simulink model "Hypnoz_embedded_continu_v008"  (Simulink 7.7)
settings: Solver=ode3  StartTime=0.0  StopTime=50  FixedStep=Ts  RelTol=1e-3
values from neighbouring files (symbols this model uses):
  A = [-r/L -k/L;km/J -lambda/J]    [SimulationParams.m]
  B = [1/L;0]    [SimulationParams.m]
  Coeff_reprise_obs_I = 1    [SimulationParams.m]
  Coeff_reprise_obs_U = 1    [SimulationParams.m]
  Cs = 196/4    (= 49)    [SimulationParams.m]
  Delt_I2t_max = 1000    [SimulationParams.m]
  Delt_Imot_max = 5    [SimulationParams.m]
  Delt_U2t_max = 1000    [SimulationParams.m]
  Delt_Umot_max = 5    [SimulationParams.m]
  I2t_max = 200000    [SimulationParams.m]
  Imot_max = 220    [SimulationParams.m]
  Isc_max = 300    [SimulationParams.m]
  k = 1/52    (= 0.0192307692308)    [SimulationParams.m]
  Ka = place(Aa,Ba,[p1 p2 p3])    [SimulationParams.m]
  km = 0.16    [SimulationParams.m]
  Koi = K(3:4,:)    [SimulationParams.m]
  Kop = K(1:2,:)    [SimulationParams.m]
  L = 53E-6    (= 5.3e-05)    [SimulationParams.m]
  Masse_vehicule = 850    [SimulationParams.m]
  Pmax_boost = 11750    [SimulationParams.m]
  Pmax_brake = 25000    [SimulationParams.m]
  r = 0.0175    [SimulationParams.m]
  rapport_vitesses = empatement/Rayon_braquage    (= 0.15)    [SimulationParams.m]
  rayon_roue = 0.31    [SimulationParams.m]
  Reduction_electrique = 1/3    (= 0.333333333333)    [SimulationParams.m]
  Th_down = -5    [SimulationParams.m]
  Th_up = 90    [SimulationParams.m]
  to = 0.03    [SimulationParams.m]
  Tr1 = 1000    [SimulationParams.m]
  Tr2 = 1000    [SimulationParams.m]
  Tr6 = 1/Ts    (= 1000)    [SimulationParams.m]
  Ts = 0.001    [SimulationParams.m]
  Ts_sc = 0.005    [SimulationParams.m]
  Umot_max = 96    [SimulationParams.m]
  Usc_max = 192    [SimulationParams.m]
  Usc_min = 96    [SimulationParams.m]
undefined symbols (not defined in the file or in its folder): sigbuilder_block
libraries: simulink x10, simulink_extras x1
(part 1 of 2)
settings Model: Creator=F.NICOLAS  LastModifiedBy=Guilherme  BufferReuse=off
settings DataIOCC: SaveOutput=off  SignalLogging=off  SaveTime=off
settings OptimizationCC: BlockReduction=off  BooleanDataType=off  OptimizeBlockIOStorage=off  BufferReuse=off  ExpressionFolding=off  LocalBlockOutputs=off  InitFltsAndDblsToZero=on
settings DebuggingCC: ArtificialAlgebraicLoopMsg=error  SaveWithParameterizedLinksMsg=none  SignalResolutionControl=TryResolveAllWithWarning  MultiTaskCondExecSysMsg=none  StrictBusMsg=Warning
settings HardwareCC: ProdHWDeviceType=Generic->Unspecified (assume 32-bit Generic)
settings SFSimCC: SimParseCustomCode=off
settings RTWCC: IncludeERTFirstTime=on
settings GRTTargetCC: TargetFcnLib=ansi_tfl_tmw.mat

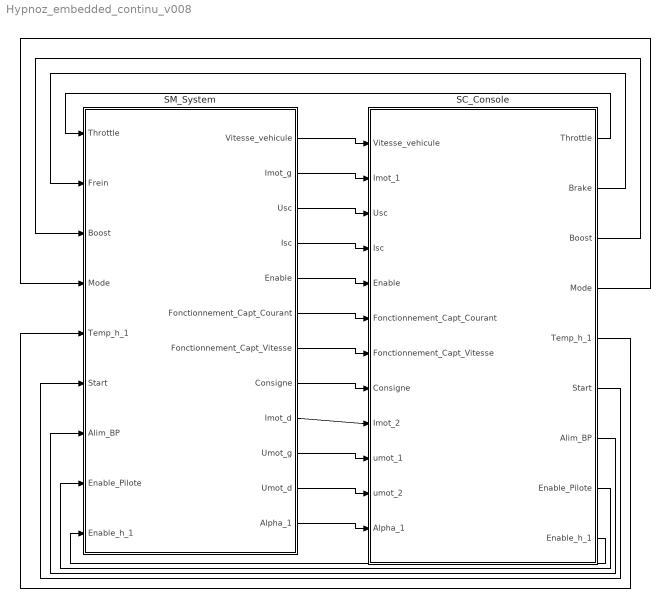
== system Hypnoz_embedded_continu_v008 ==
  SC_Console : Subsystem
  SM_System : Subsystem
  wires:
  SC_Console/1(Throttle) -> SM_System/1(Throttle)
  SC_Console/3(Boost) -> SM_System/3(Boost)
  SM_System/1(Vitesse_vehicule) -> SC_Console/1(Vitesse_vehicule)
  SC_Console/4(Mode) -> SM_System/4(Mode)
  SC_Console/2(Brake) -> SM_System/2(Frein)
  SM_System/2(Imot_g) -> SC_Console/2(Imot_1)
  SM_System/3(Usc) -> SC_Console/3(Usc)
  SM_System/4(Isc) -> SC_Console/4(Isc)
  SM_System/5(Enable) -> SC_Console/5(Enable)
  SM_System/6(Fonctionnement_Capt_Courant) -> SC_Console/6(Fonctionnement_Capt_Courant)
  SM_System/8(Consigne) -> SC_Console/8(Consigne)
  SM_System/9(Imot_d) -> SC_Console/9(Imot_2)
  SM_System/10(Umot_g) -> SC_Console/10(umot_1)
  SM_System/11(Umot_d) -> SC_Console/11(umot_2)
  SM_System/7(Fonctionnement_Capt_Vitesse) -> SC_Console/7(Fonctionnement_Capt_Vitesse)
  SC_Console/9(Enable_h_1) -> SM_System/9(Enable_h_1)
  SC_Console/8(Enable_Pilote) -> SM_System/8(Enable_Pilote)
  SC_Console/7(Alim_BP) -> SM_System/7(Alim_BP)
  SC_Console/6(Start) -> SM_System/6(Start)
  SC_Console/5(Temp_h_1) -> SM_System/5(Temp_h_1)
  SM_System/12(Alpha_1) -> SC_Console/12(Alpha_1)

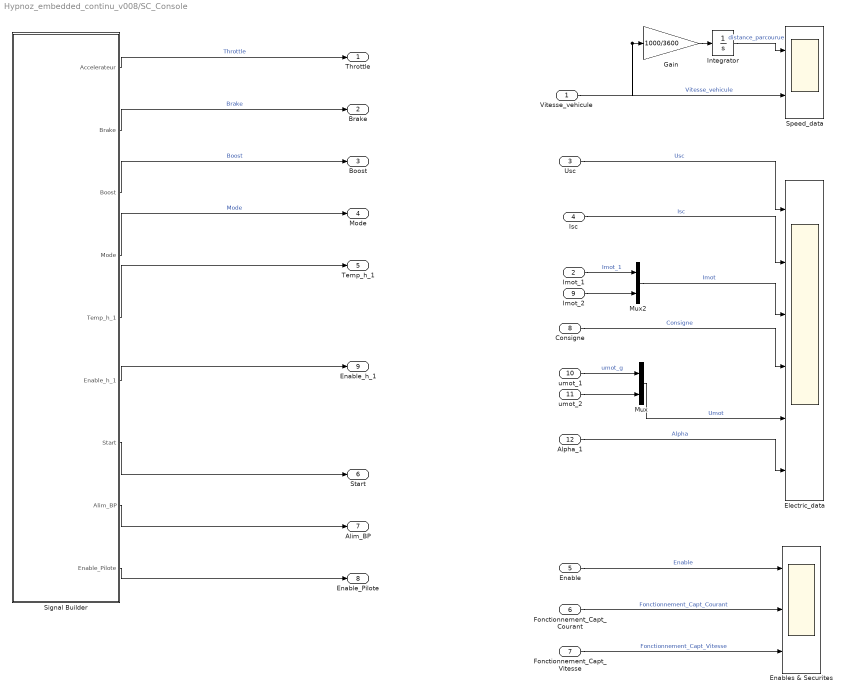
== system Hypnoz_embedded_continu_v008/SC_Console ==
  Vitesse_vehicule : Inport
  Imot_1 : Inport  Port=2
  Usc : Inport  Port=3
  Isc : Inport  Port=4
  Enable : Inport  Port=5
  Fonctionnement_Capt_Courant : Inport  Port=6
  Fonctionnement_Capt_Vitesse : Inport  Port=7
  Consigne : Inport  Port=8
  Imot_2 : Inport  Port=9
  umot_1 : Inport  Port=10
  umot_2 : Inport  Port=11
  Alpha_1 : Inport  Port=12
  Electric_data : Scope  NumInputPorts=6
      settings: TimeRange=4  YMin=149.1~-9~55~0~0.5~0.01  YMax=150~-1~100~100~5~0.045  SaveName=ScopeData21
  Enables & Securites : Scope  NumInputPorts=3
      settings: YMin=0.95~0.95~0.95  YMax=1.05~1.05~1.05
  Gain : Gain  Gain=1000/3600
  Integrator : Integrator
  Mux : Mux  Inputs=2
  Mux2 : Mux  Inputs=2
  Signal Builder : Subsystem  Tag=STV Subsys  LoadFcn=sigbuilder_block('load');  StartFcn=sigbuilder_block('start');  StopFcn=sigbuilder_block('stop');  ClipboardFcn=sigbuilder_block('clipboard');  mask(Sigbuilder block){}
      mask help: Sigbuilder GUI
      mask init:
      | if ~strcmp(get_param(bdroot(gcbh),'SimulationStatus'),'stopped') tuvar = sigbuilder_block('maskInit'); end
      settings: CopyFcn=sigbuilder_block('copy');  DeleteFcn=sigbuilder_block('delete');  ModelCloseFcn=sigbuilder_block('modelClose');  PreSaveFcn=sigbuilder_block('preSave');  NameChangeFcn=sigbuilder_block('namechange');  OpenFcn=sigbuilder_block('open',[6 21 1012.5 492 ]);  CloseFcn=sigbuilder_block('close');
      mask Display: plot(0,0,100,100,[10,10,40,40,10],[80,20,20,80,80],[40,10],[50,50], [40,27,10],[65,72,56],[40,25,25,10],[28,28,43,43]);
  Speed_data : Scope  NumInputPorts=2
      settings: TimeRange=4  YMin=10~27.5  YMax=90~52.5
  Throttle : Outport
  Brake : Outport  Port=2
  Boost : Outport  Port=3
  Mode : Outport  Port=4
  Temp_h_1 : Outport  Port=5
  Start : Outport  Port=6
  Alim_BP : Outport  Port=7
  Enable_Pilote : Outport  Port=8
  Enable_h_1 : Outport  Port=9
  wires:
  Signal Builder/1(Accelerateur) -> Throttle/1  "Throttle"
  Vitesse_vehicule/1 -> Gain/1, Speed_data/2  "Vitesse_vehicule"
  Signal Builder/2(Brake) -> Brake/1  "Brake"
  Signal Builder/3(Boost) -> Boost/1  "Boost"
  Signal Builder/4(Mode) -> Mode/1  "Mode"
  Gain/1 -> Integrator/1
  Integrator/1 -> Speed_data/1  "distance_parcourue"
  Usc/1 -> Electric_data/1  "Usc"
  Isc/1 -> Electric_data/2  "Isc"
  Signal Builder/5(Temp_h_1) -> Temp_h_1/1
  Consigne/1 -> Electric_data/4  "Consigne"
  Signal Builder/6(Enable_h_1) -> Enable_h_1/1
  Signal Builder/7(Start) -> Start/1
  Signal Builder/8(Alim_BP) -> Alim_BP/1
  Signal Builder/9(Enable_Pilote) -> Enable_Pilote/1
  Imot_1/1 -> Mux2/1  "Imot_1"
  Enable/1 -> Enables & Securites/1  "Enable"
  Fonctionnement_Capt_Courant/1 -> Enables & Securites/2  "Fonctionnement_Capt_Courant"
  Fonctionnement_Capt_Vitesse/1 -> Enables & Securites/3  "Fonctionnement_Capt_Vitesse"
  Mux/1 -> Electric_data/5  "Umot"
  umot_1/1 -> Mux/1  "umot_g"
  Alpha_1/1 -> Electric_data/6  "Alpha"
  umot_2/1 -> Mux/2
  Mux2/1 -> Electric_data/3  "Imot"
  Imot_2/1 -> Mux2/2

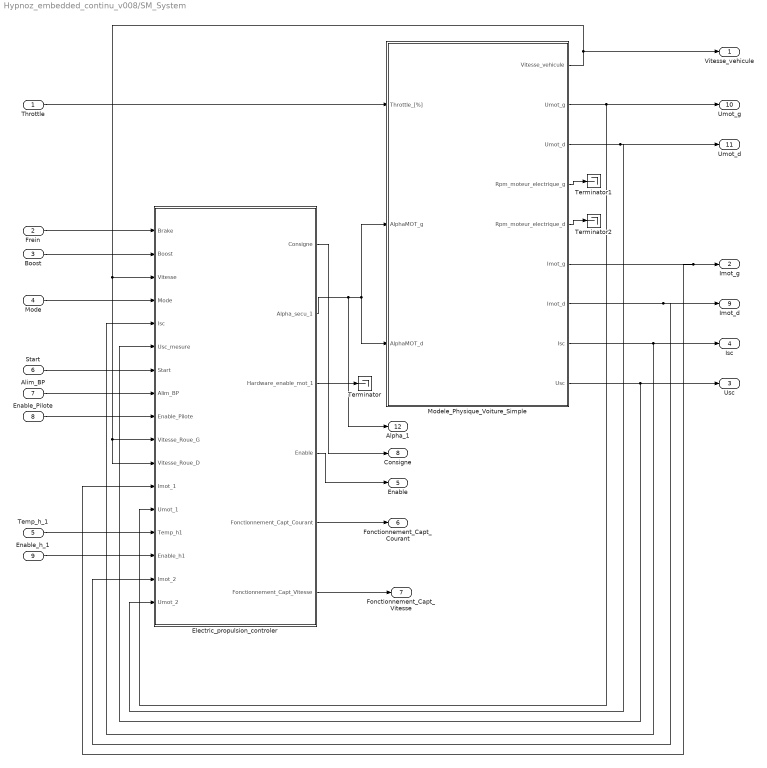
== system Hypnoz_embedded_continu_v008/SM_System ==
  Throttle : Inport
  Frein : Inport  Port=2
  Boost : Inport  Port=3
  Mode : Inport  Port=4
  Temp_h_1 : Inport  Port=5
  Start : Inport  Port=6
  Alim_BP : Inport  Port=7
  Enable_Pilote : Inport  Port=8
  Enable_h_1 : Inport  Port=9
  Electric_propulsion_controler : Subsystem
  Modele_Physique_Voiture_Simple : Subsystem
  Terminator : Terminator
  Terminator1 : Terminator
  Terminator2 : Terminator
  Vitesse_vehicule : Outport
  Imot_g : Outport  Port=2
  Usc : Outport  Port=3
  Isc : Outport  Port=4
  Enable : Outport  Port=5
  Fonctionnement_Capt_Courant : Outport  Port=6
  Fonctionnement_Capt_Vitesse : Outport  Port=7
  Consigne : Outport  Port=8
  Imot_d : Outport  Port=9
  Umot_g : Outport  Port=10
  Umot_d : Outport  Port=11
  Alpha_1 : Outport  Port=12
  wires:
  Modele_Physique_Voiture_Simple/1(Vitesse_vehicule) -> Vitesse_vehicule/1, Electric_propulsion_controler/3(Vitesse), Electric_propulsion_controler/10(Vitesse_Roue_G), Electric_propulsion_controler/11(Vitesse_Roue_D)
  Boost/1 -> Electric_propulsion_controler/2(Boost)
  Mode/1 -> Electric_propulsion_controler/4(Mode)
  Electric_propulsion_controler/4(Enable) -> Enable/1
  Electric_propulsion_controler/1(Consigne) -> Consigne/1
  Modele_Physique_Voiture_Simple/6(Imot_g) -> Imot_g/1, Electric_propulsion_controler/12(Imot_1)
  Modele_Physique_Voiture_Simple/7(Imot_d) -> Imot_d/1, Electric_propulsion_controler/16(Imot_2)
  Modele_Physique_Voiture_Simple/8(Isc) -> Isc/1, Electric_propulsion_controler/5(Isc)
  Frein/1 -> Electric_propulsion_controler/1(Brake)
  Modele_Physique_Voiture_Simple/9(Usc) -> Usc/1, Electric_propulsion_controler/6(Usc_mesure)
  Modele_Physique_Voiture_Simple/3(Umot_d) -> Umot_d/1, Electric_propulsion_controler/17(Umot_2)
  Modele_Physique_Voiture_Simple/2(Umot_g) -> Umot_g/1, Electric_propulsion_controler/13(Umot_1)
  Electric_propulsion_controler/2(Alpha_secu_1) -> Alpha_1/1, Modele_Physique_Voiture_Simple/2(AlphaMOT_g), Modele_Physique_Voiture_Simple/3(AlphaMOT_d)
  Electric_propulsion_controler/5(Fonctionnement_Capt_Courant) -> Fonctionnement_Capt_Courant/1
  Electric_propulsion_controler/6(Fonctionnement_Capt_Vitesse) -> Fonctionnement_Capt_Vitesse/1
  Temp_h_1/1 -> Electric_propulsion_controler/14(Temp_h1)
  Start/1 -> Electric_propulsion_controler/7(Start)
  Alim_BP/1 -> Electric_propulsion_controler/8(Alim_BP)
  Enable_Pilote/1 -> Electric_propulsion_controler/9(Enable_Pilote)
  Enable_h_1/1 -> Electric_propulsion_controler/15(Enable_h1)
  Throttle/1 -> Modele_Physique_Voiture_Simple/1(Throttle_[%])
  Electric_propulsion_controler/3(Hardware_enable_mot_1) -> Terminator/1
  Modele_Physique_Voiture_Simple/4(Rpm_moteur_electrique_g) -> Terminator1/1
  Modele_Physique_Voiture_Simple/5(Rpm_moteur_electrique_d) -> Terminator2/1

== system Hypnoz_embedded_continu_v008/SC_Console/Signal Builder ==
  Demux : Demux  Tag=STV Demux  Outputs=9
  FromWs : FromWorkspace  Tag=STV FromWs  VariableName=tuvar  SampleTime=0  SigBuilderData=DataTag0  VnvData=DataTag1
      SigBuilderData=|
      | common.afterFinalStr = 'Extrapolate'
      | common.sampleTime = 0
      | dataSet.timeRange = [0 40]
      | dataSet.name = 'Group 1'
      | sbobj.Groups(1).Name = 'Group 1'
      | sbobj.Groups(1).Signals(1).Name = 'Accelerateur'
      | sbobj.Groups(1).Signals(1).XData = [0 40]
      | sbobj.Groups(1).Signals(1).YData = [0 0]
      | sbobj.Groups(1).Signals(2).Name = 'Brake'
      | sbobj.Groups(1).Signals(2).XData = [0 1.57 2.48 5.39 5.82 20 20 30 30 40]
      | sbobj.Groups(1).Signals(2).YData = [0 0 0 0 0 0 0.95 0.95 0 0]
      | sbobj.Groups(1).Signals(3).Name = 'Boost'
      | sbobj.Groups(1).Signals(3).XData = [0 5 10 15 15 20 25 30 35 40]
      | sbobj.Groups(1).Signals(3).YData = [0 0 1 1 0 0 0 0 0 0]
      | sbobj.Groups(1).Signals(4).Name = 'Mode'
      | sbobj.Groups(1).Signals(4).XData = [0 40]
      | sbobj.Groups(1).Signals(4).YData = [2 2]
      | sbobj.Groups(1).Signals(5).Name = 'Temp_h_1'
      | sbobj.Groups(1).Signals(5).XData = [0 40]
      | sbobj.Groups(1).Signals(5).YData = [60 60]
      | sbobj.Groups(1).Signals(6).Name = 'Enable_h_1'
      | sbobj.Groups(1).Signals(6).XData = [0 40]
      | sbobj.Groups(1).Signals(6).YData = [1 1]
      | sbobj.Groups(1).Signals(7).Name = 'Start'
      | sbobj.Groups(1).Signals(7).XData = [0 1 1 2 2 40]
      | sbobj.Groups(1).Signals(7).YData = [0 0 1 1 0 0]
      | sbobj.Groups(1).Signals(8).Name = 'Alim_BP'
      | sbobj.Groups(1).Signals(8).XData = [0 40]
      | sbobj.Groups(1).Signals(8).YData = [1 1]
      | sbobj.Groups(1).Signals(9).Name = 'Enable_Pilote'
      | sbobj.Groups(1).Signals(9).XData = [0 40]
      | sbobj.Groups(1).Signals(9).YData = [1 1]
      | sbobj.Groups(1).TimeRange = [0 40]
      | sbobj.Groups(2).Name = 'Group 2'
      | sbobj.Groups(2).Signals(1).Name = 'Accelerateur'
      | sbobj.Groups(2).Signals(1).XData = [0 100]
      | sbobj.Groups(2).Signals(1).YData = [0 0]
      | sbobj.Groups(2).Signals(2).Name = 'Brake'
      | sbobj.Groups(2).Signals(2).XData = [0 1.57 2.48 5.39 5.82 19.1 27.1 100]
      | sbobj.Groups(2).Signals(2).YData = [0 0 0 0 0 0 0 0]
      | sbobj.Groups(2).Signals(3).Name = 'Boost'
      | sbobj.Groups(2).Signals(3).XData = [0 10 20 20 30 30 40 40 50 50 60 60 70 70 80 80 90 90 100]
      | sbobj.Groups(2).Signals(3).YData = [0 0 2 0 2 0 2 0 2 0 2 0 2 0 2 0 2 0 2]
      | sbobj.Groups(2).Signals(4).Name = 'Mode'
      | sbobj.Groups(2).Signals(4).XData = [0 100]
      | sbobj.Groups(2).Signals(4).YData = [2 2]
      | sbobj.Groups(2).Signals(5).Name = 'Temp_h_1'
      | sbobj.Groups(2).Signals(5).XData = [0 100]
      | sbobj.Groups(2).Signals(5).YData = [60 60]
      | sbobj.Groups(2).Signals(6).Name = 'Enable_h_1'
      | sbobj.Groups(2).Signals(6).XData = [0 100]
      | sbobj.Groups(2).Signals(6).YData = [1 1]
      | sbobj.Groups(2).Signals(7).Name = 'Start'
      | sbobj.Groups(2).Signals(7).XData = [0 1 1 2 2 100]
      | sbobj.Groups(2).Signals(7).YData = [0 0 1 1 0 0]
      | sbobj.Groups(2).Signals(8).Name = 'Alim_BP'
      | sbobj.Groups(2).Signals(8).XData = [0 100]
      | sbobj.Groups(2).Signals(8).YData = [1 1]
      | sbobj.Groups(2).Signals(9).Name = 'Enable_Pilote'
      | sbobj.Groups(2).Signals(9).XData = [0 100]
      | sbobj.Groups(2).Signals(9).YData = [1 1]
  Accelerateur : Outport  Tag=STV Outport
  Brake : Outport  Tag=STV Outport  Port=2
  Boost : Outport  Tag=STV Outport  Port=3
  Mode : Outport  Tag=STV Outport  Port=4
  Temp_h_1 : Outport  Tag=STV Outport  Port=5
  Enable_h_1 : Outport  Tag=STV Outport  Port=6
  Start : Outport  Tag=STV Outport  Port=7
  Alim_BP : Outport  Tag=STV Outport  Port=8
  Enable_Pilote : Outport  Tag=STV Outport  Port=9
  wires:
  FromWs/1 -> Demux/1
  Demux/1 -> Accelerateur/1
  Demux/2 -> Brake/1
  Demux/3 -> Boost/1
  Demux/4 -> Mode/1
  Demux/5 -> Temp_h_1/1
  Demux/6 -> Enable_h_1/1
  Demux/7 -> Start/1
  Demux/8 -> Alim_BP/1
  Demux/9 -> Enable_Pilote/1

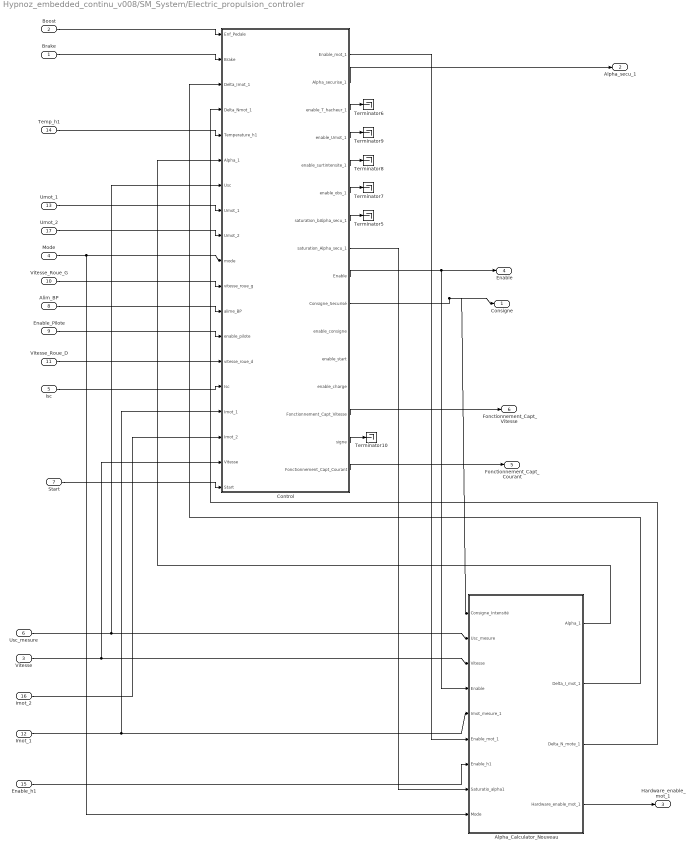
== system Hypnoz_embedded_continu_v008/SM_System/Electric_propulsion_controler ==
  Brake : Inport
  Boost : Inport  Port=2
  Vitesse : Inport  Port=3
  Mode : Inport  Port=4
  Isc : Inport  Port=5
  Usc_mesure : Inport  Port=6
  Start : Inport  Port=7
  Alim_BP : Inport  Port=8
  Enable_Pilote : Inport  Port=9
  Vitesse_Roue_G : Inport  Port=10
  Vitesse_Roue_D : Inport  Port=11
  Imot_1 : Inport  Port=12
  Umot_1 : Inport  Port=13
  Temp_h1 : Inport  Port=14
  Enable_h1 : Inport  Port=15
  Imot_2 : Inport  Port=16
  Umot_2 : Inport  Port=17
  Alpha_Calculator_Nouveau : Subsystem
  Control : Subsystem
  Terminator{5..10} (6 alike) : Terminator
  Consigne : Outport
  Alpha_secu_1 : Outport  Port=2
  Hardware_enable_mot_1 : Outport  Port=3
  Enable : Outport  Port=4
  Fonctionnement_Capt_Courant : Outport  Port=5
  Fonctionnement_Capt_Vitesse : Outport  Port=6
  wires:
  Control/10(Consigne_Securisé) -> Alpha_Calculator_Nouveau/1(Consigne_Intensité), Consigne/1
  Alpha_Calculator_Nouveau/1(Alpha_1) -> Control/6(Alpha_1)
  Boost/1 -> Control/1(Enf_Pedale)
  Brake/1 -> Control/2(Brake)
  Control/9(Enable) -> Alpha_Calculator_Nouveau/4(Enable), Enable/1
  Control/1(Enable_mot_1) -> Alpha_Calculator_Nouveau/6(Enable_mot_1)
  Mode/1 -> Control/10(mode), Alpha_Calculator_Nouveau/9(Mode)
  Usc_mesure/1 -> Alpha_Calculator_Nouveau/2(Usc_mesure), Control/7(Usc)
  Imot_1/1 -> Alpha_Calculator_Nouveau/5(Imot_mesure_1), Control/16(Imot_1)
  Imot_2/1 -> Control/17(Imot_2)
  Isc/1 -> Control/15(Isc)
  Vitesse/1 -> Alpha_Calculator_Nouveau/3(Vitesse), Control/18(Vitesse)
  Enable_h1/1 -> Alpha_Calculator_Nouveau/7(Enable_h1)
  Control/8(saturation_Alpha_secu_1) -> Alpha_Calculator_Nouveau/8(Saturatio_alpha1)
  Control/7(saturation_bAlpha_secu_1) -> Terminator5/1
  Control/6(enable_obs_1) -> Terminator7/1
  Control/5(enable_surtintensite_1) -> Terminator8/1
  Control/4(enable_Umot_1) -> Terminator9/1
  Control/3(enable_T_hacheur_1) -> Terminator6/1
  Temp_h1/1 -> Control/5(Temperature_h1)
  Umot_2/1 -> Control/9(Umot_2)
  Umot_1/1 -> Control/8(Umot_1)
  Vitesse_Roue_D/1 -> Control/14(vitesse_roue_d)
  Vitesse_Roue_G/1 -> Control/11(vitesse_roue_g)
  Start/1 -> Control/19(Start)
  Enable_Pilote/1 -> Control/13(enable_pilote)
  Alim_BP/1 -> Control/12(alime_BP)
  Alpha_Calculator_Nouveau/2(Delta_I_mot_1) -> Control/3(Delta_Imot_1)
  Alpha_Calculator_Nouveau/3(Delta_N_mote_1) -> Control/4(Delta_Nmot_1)
  Control/2(Alpha_securise_1) -> Alpha_secu_1/1
  Alpha_Calculator_Nouveau/4(Hardware_enable_mot_1) -> Hardware_enable_mot_1/1
  Control/16(Fonctionnement_Capt_Courant) -> Fonctionnement_Capt_Courant/1
  Control/14(Fonctionnement_Capt_Vitesse) -> Fonctionnement_Capt_Vitesse/1
  Control/15(signe) -> Terminator10/1

== system Hypnoz_embedded_continu_v008/SM_System/Modele_Physique_Voiture_Simple ==
  Throttle_[%] : Inport
  AlphaMOT_g : Inport  Port=2
  AlphaMOT_d : Inport  Port=3
  Circuit_electrique_HP : Subsystem
  Couple_Max : Gain  Gain=130
  Modèle_Simplifiè Véhicule : Subsystem
  Terminator : Terminator
  Vitesse_vehicule : Outport
  Umot_g : Outport  Port=2
  Umot_d : Outport  Port=3
  Rpm_moteur_electrique_g : Outport  Port=4
  Rpm_moteur_electrique_d : Outport  Port=5
  Imot_g : Outport  Port=6
  Imot_d : Outport  Port=7
  Isc : Outport  Port=8
  Usc : Outport  Port=9
  wires:
  Circuit_electrique_HP/2(I Mot_d) -> Imot_d/1, Modèle_Simplifiè Véhicule/3(Imot_d)
  AlphaMOT_g/1 -> Circuit_electrique_HP/3(AlphaMOT_g)
  AlphaMOT_d/1 -> Circuit_electrique_HP/4(AlphaMOT_d)
  Circuit_electrique_HP/3(Isc) -> Isc/1
  Circuit_electrique_HP/4(Usc) -> Usc/1
  Circuit_electrique_HP/5(Umot_g) -> Umot_g/1
  Circuit_electrique_HP/6(Umot_d) -> Umot_d/1
  Circuit_electrique_HP/1(I Mot_g) -> Imot_g/1, Modèle_Simplifiè Véhicule/2(Imot_g)
  Throttle_[%]/1 -> Couple_Max/1
  Couple_Max/1 -> Modèle_Simplifiè Véhicule/1(Couple_thermique)
  Modèle_Simplifiè Véhicule/2(Vitesse_Vehicule) -> Vitesse_vehicule/1
  Modèle_Simplifiè Véhicule/3(RPM_Moteur_Electrique) -> Rpm_moteur_electrique_g/1, Circuit_electrique_HP/1(Rpm_moteur_electrique_g), Rpm_moteur_electrique_d/1, Circuit_electrique_HP/2(Rpm_moteur_electrique_d)
  Modèle_Simplifiè Véhicule/1(couple_roue) -> Terminator/1

== system Hypnoz_embedded_continu_v008/SM_System/Electric_propulsion_controler/Alpha_Calculator_Nouveau ==
  Consigne_Intensité : Inport
  Usc_mesure : Inport  Port=2
  Vitesse : Inport  Port=3
  Enable : Inport  Port=4
  Imot_mesure_1 : Inport  Port=5
  Enable_mot_1 : Inport  Port=6
  Enable_h1 : Inport  Port=7
  Saturatio_alpha1 : Inport  Port=8
  Mode : Inport  Port=9
  Alpha_calculator_motg1 : Subsystem
  Alpha_1 : Outport
  Delta_I_mot_1 : Outport  Port=2
  Delta_N_mote_1 : Outport  Port=3
  Hardware_enable_mot_1 : Outport  Port=4
  wires:
  Consigne_Intensité/1 -> Alpha_calculator_motg1/1(Consigne_intensité)
  Alpha_calculator_motg1/1(Alpha_g) -> Alpha_1/1
  Imot_mesure_1/1 -> Alpha_calculator_motg1/2(Imot_mesure_g)
  Usc_mesure/1 -> Alpha_calculator_motg1/3(Usc_mesure)
  Alpha_calculator_motg1/2(Delta_I_mot_g1) -> Delta_I_mot_1/1
  Vitesse/1 -> Alpha_calculator_motg1/4(Vitesse)
  Enable/1 -> Alpha_calculator_motg1/5(enable)
  Enable_mot_1/1 -> Alpha_calculator_motg1/6(enable_mot_g1)
  Alpha_calculator_motg1/3(Delta_N_mot_g1) -> Delta_N_mote_1/1
  Saturatio_alpha1/1 -> Alpha_calculator_motg1/8(Saturation_alpha1)
  Alpha_calculator_motg1/4(Hardware_enable_mot_1) -> Hardware_enable_mot_1/1
  Enable_h1/1 -> Alpha_calculator_motg1/7(enable_h1)
  Mode/1 -> Alpha_calculator_motg1/9(mode)

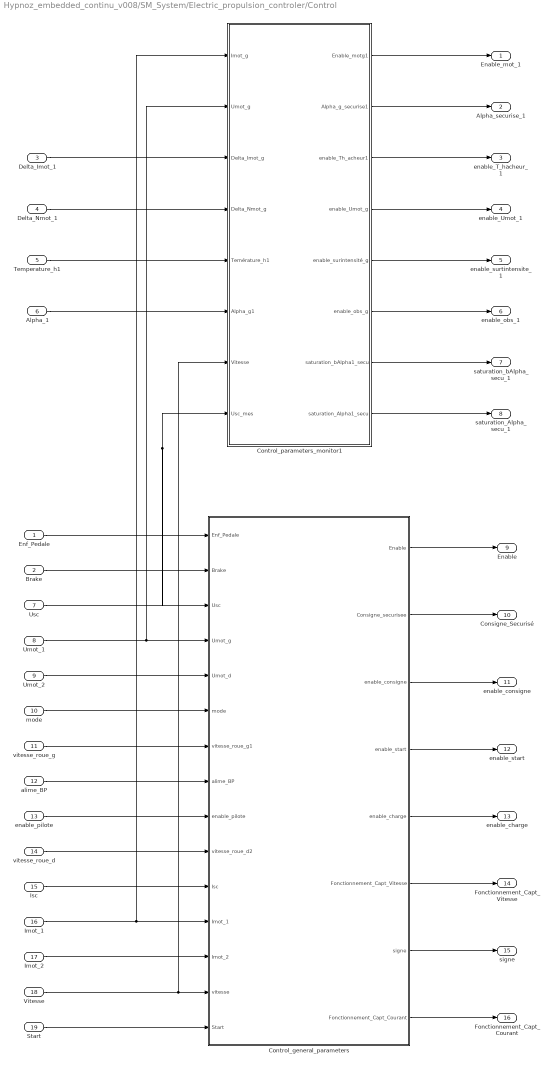
== system Hypnoz_embedded_continu_v008/SM_System/Electric_propulsion_controler/Control ==
  Enf_Pedale : Inport
  Brake : Inport  Port=2
  Delta_Imot_1 : Inport  Port=3
  Delta_Nmot_1 : Inport  Port=4
  Temperature_h1 : Inport  Port=5
  Alpha_1 : Inport  Port=6
  Usc : Inport  Port=7
  Umot_1 : Inport  Port=8
  Umot_2 : Inport  Port=9
  mode : Inport  Port=10
  vitesse_roue_g : Inport  Port=11
  alime_BP : Inport  Port=12
  enable_pilote : Inport  Port=13
  vitesse_roue_d : Inport  Port=14
  Isc : Inport  Port=15
  Imot_1 : Inport  Port=16
  Imot_2 : Inport  Port=17
  Vitesse : Inport  Port=18
  Start : Inport  Port=19
  Control_general_parameters : Subsystem
  Control_parameters_monitor1 : Subsystem
  Enable_mot_1 : Outport
  Alpha_securise_1 : Outport  Port=2
  enable_T_hacheur_1 : Outport  Port=3
  enable_Umot_1 : Outport  Port=4
  enable_surtintensite_1 : Outport  Port=5
  enable_obs_1 : Outport  Port=6
  saturation_bAlpha_secu_1 : Outport  Port=7
  saturation_Alpha_secu_1 : Outport  Port=8
  Enable : Outport  Port=9
  Consigne_Securisé : Outport  Port=10
  enable_consigne : Outport  Port=11
  enable_start : Outport  Port=12
  enable_charge : Outport  Port=13
  Fonctionnement_Capt_Vitesse : Outport  Port=14
  signe : Outport  Port=15
  Fonctionnement_Capt_Courant : Outport  Port=16
  wires:
  Control_general_parameters/1(Enable) -> Enable/1
  Brake/1 -> Control_general_parameters/2(Brake)
  Control_general_parameters/2(Consigne_securisee) -> Consigne_Securisé/1
  Umot_1/1 -> Control_general_parameters/4(Umot_g), Control_parameters_monitor1/2(Umot_g)
  Umot_2/1 -> Control_general_parameters/5(Umot_d)
  Control_general_parameters/3(enable_consigne) -> enable_consigne/1
  mode/1 -> Control_general_parameters/6(mode)
  vitesse_roue_g/1 -> Control_general_parameters/7(vitesse_roue_g1)
  Control_general_parameters/4(enable_start) -> enable_start/1
  alime_BP/1 -> Control_general_parameters/8(alime_BP)
  enable_pilote/1 -> Control_general_parameters/9(enable_pilote)
  Control_general_parameters/5(enable_charge) -> enable_charge/1
  vitesse_roue_d/1 -> Control_general_parameters/10(vitesse_roue_d2)
  Control_general_parameters/6(Fonctionnement_Capt_Vitesse) -> Fonctionnement_Capt_Vitesse/1
  Isc/1 -> Control_general_parameters/11(Isc)
  Imot_1/1 -> Control_general_parameters/12(Imot_1), Control_parameters_monitor1/1(Imot_g)
  Control_general_parameters/7(signe) -> signe/1
  Imot_2/1 -> Control_general_parameters/13(Imot_2)
  Control_general_parameters/8(Fonctionnement_Capt_Courant) -> Fonctionnement_Capt_Courant/1
  Start/1 -> Control_general_parameters/15(Start)
  Vitesse/1 -> Control_general_parameters/14(vitesse), Control_parameters_monitor1/7(Vitesse)
  Control_parameters_monitor1/1(Enable_motg1) -> Enable_mot_1/1
  Control_parameters_monitor1/2(Alpha_g_securise1) -> Alpha_securise_1/1
  Delta_Imot_1/1 -> Control_parameters_monitor1/3(Delta_Imot_g)
  Control_parameters_monitor1/3(enable_Th_acheur1) -> enable_T_hacheur_1/1
  Delta_Nmot_1/1 -> Control_parameters_monitor1/4(Delta_Nmot_g)
  Control_parameters_monitor1/4(enable_Umot_g) -> enable_Umot_1/1
  Temperature_h1/1 -> Control_parameters_monitor1/5(Temérature_h1)
  Control_parameters_monitor1/5(enable_surintensité_g) -> enable_surtintensite_1/1
  Alpha_1/1 -> Control_parameters_monitor1/6(Alpha_g1)
  Control_parameters_monitor1/6(enable_obs_g) -> enable_obs_1/1
  Control_parameters_monitor1/7(saturation_bAlpha1_secu) -> saturation_bAlpha_secu_1/1
  Usc/1 -> Control_parameters_monitor1/8(Usc_mes), Control_general_parameters/3(Usc)
  Control_parameters_monitor1/8(saturation_Alpha1_secu) -> saturation_Alpha_secu_1/1
  Enf_Pedale/1 -> Control_general_parameters/1(" Enf_Pedale")

== system Hypnoz_embedded_continu_v008/SM_System/Modele_Physique_Voiture_Simple/Circuit_electrique_HP ==
  Rpm_moteur_electrique_g : Inport
  Rpm_moteur_electrique_d : Inport  Port=2
  AlphaMOT_g : Inport  Port=3
  AlphaMOT_d : Inport  Port=4
  Add6 : Sum  Inputs=--
  Moteur_electrique_d : Subsystem
  Moteur_electrique_g : Subsystem
  Product{,1..3} (4 alike) : Product  RndMeth=Zero
  Scope : Scope  NumInputPorts=2
      settings: YMin=-5~-5  YMax=5~5  SaveName=ScopeData28
  Supercapas1 : simulink_extras/Additional Linear/Transfer Fcn (with initial states)  SystemSampleTime=-1  N=[1]  D=[Cs 0]  X0=150*Cs
  V_to_U_d : Gain  Gain=k
  V_to_U_g : Gain  Gain=k
  I Mot_g : Outport
  I Mot_d : Outport  Port=2
  Isc : Outport  Port=3
  Usc : Outport  Port=4
  Umot_g : Outport  Port=5
  Umot_d : Outport  Port=6
  wires:
  Moteur_electrique_g/1(CourantMoteur) -> I Mot_g/1, Product/2
  Rpm_moteur_electrique_g/1 -> Moteur_electrique_g/2(Vitesse), V_to_U_g/1
  AlphaMOT_g/1 -> Product/1, Scope/1, Product3/1
  V_to_U_g/1 -> Umot_g/1
  Product/1 -> Add6/1
  Moteur_electrique_d/1(CourantMoteur) -> I Mot_d/1, Product2/2
  Rpm_moteur_electrique_d/1 -> Moteur_electrique_d/2(Vitesse), V_to_U_d/1
  AlphaMOT_d/1 -> Product2/1, Product1/2
  V_to_U_d/1 -> Umot_d/1
  Product2/1 -> Add6/2
  Add6/1 -> Supercapas1/1, Isc/1
  Supercapas1/1 -> Usc/1, Product1/1, Product3/2
  Product1/1 -> Moteur_electrique_d/1(TensionSortieHacheur)
  Product3/1 -> Moteur_electrique_g/1(TensionSortieHacheur), Scope/2

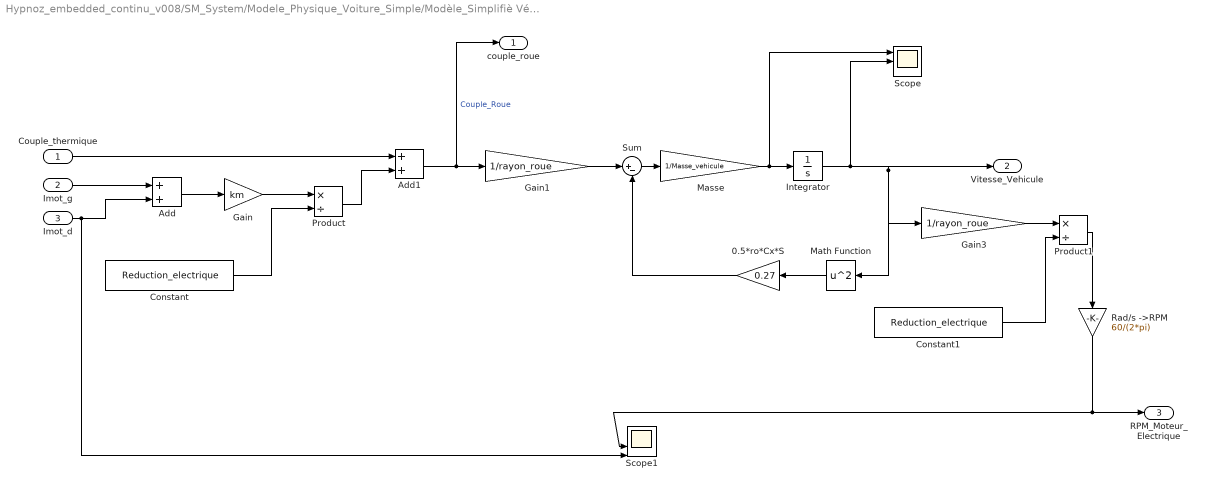
== system Hypnoz_embedded_continu_v008/SM_System/Modele_Physique_Voiture_Simple/Modèle_Simplifiè Véhicule ==
  Couple_thermique : Inport
  Imot_g : Inport  Port=2
  Imot_d : Inport  Port=3
  0.5*ro*Cx*S : Gain  Gain=0.27
  Add : Sum
  Add1 : Sum
  Constant : Constant  Value=Reduction_electrique
  Constant1 : Constant  Value=Reduction_electrique
  Gain : Gain  Gain=km
  Gain1 : Gain  Gain=1/rayon_roue
  Gain3 : Gain  Gain=1/rayon_roue
  Integrator : Integrator
  Masse : Gain  Gain=1/Masse_vehicule
  Math Function : Math  Operator=square  SaturateOnIntegerOverflow=on
  Product : Product  Inputs=*/  RndMeth=Zero
  Product1 : Product  Inputs=*/  RndMeth=Zero
  Rad/s ->RPM : Gain  Gain=60/(2*pi)
  Scope : Scope  NumInputPorts=3
      settings: TimeRange=15  YMin=-5~-5~-5  YMax=5~5~5  SaveName=ScopeData4  MaxDataPoints=50000
  Scope1 : Scope  NumInputPorts=4
      settings: YMin=-1e-046~-5~-5~-5  YMax=1.7e-045~5~5~5  SaveName=ScopeData27  MaxDataPoints=50000
  Sum : Sum  Inputs=|+-
  couple_roue : Outport
  Vitesse_Vehicule : Outport  Port=2
  RPM_Moteur_Electrique : Outport  Port=3
  wires:
  Constant/1 -> Product/2
  Product/1 -> Add1/2
  Add1/1 -> Gain1/1, couple_roue/1  "Couple_Roue"
  Imot_g/1 -> Add/1
  Imot_d/1 -> Add/2, Scope1/4
  Add/1 -> Gain/1
  Gain/1 -> Product/1
  Couple_thermique/1 -> Add1/1
  Integrator/1 -> Math Function/1, Vitesse_Vehicule/1, Gain3/1, Scope/2
  0.5*ro*Cx*S/1 -> Sum/2
  Math Function/1 -> 0.5*ro*Cx*S/1
  Constant1/1 -> Product1/2
  Product1/1 -> Rad/s ->RPM/1
  Gain1/1 -> Sum/1
  Sum/1 -> Masse/1
  Masse/1 -> Integrator/1, Scope/1
  Gain3/1 -> Product1/1
  Rad/s ->RPM/1 -> Scope1/3, RPM_Moteur_Electrique/1

== system Hypnoz_embedded_continu_v008/SM_System/Electric_propulsion_controler/Alpha_Calculator_Nouveau/Alpha_calculator_motg1 ==
  note: alpha_g
  Consigne_intensité : Inport
  Imot_mesure_g : Inport  Port=2
  Usc_mesure : Inport  Port=3
  Vitesse : Inport  Port=4
  enable : Inport  Port=5
  enable_mot_g1 : Inport  Port=6
  enable_h1 : Inport  Port=7
  Saturation_alpha1 : Inport  Port=8
  mode : Inport  Port=9
  Constant : Constant
  Data Type Conversion : DataTypeConversion
  Display : Display
  Divide : Product  Inputs=*/
  Logical Operator : Logic  Inputs=3  AllPortsSameDT=off  OutDataTypeStr=boolean
  Retour_états_moteur_g : Subsystem
  Saturation : Saturate  UpperLimit=1  LowerLimit=0
  Sum : Sum  Inputs=++|-
  detection_saturation_correcteur1 : Subsystem
  Alpha_g : Outport
  Delta_I_mot_g1 : Outport  Port=2
  Delta_N_mot_g1 : Outport  Port=3
  Hardware_enable_mot_1 : Outport  Port=4
  wires:
  Vitesse/1 -> Retour_états_moteur_g/3(Vitesse_g)
  Retour_états_moteur_g/1(Umot_consigne_g) -> Divide/1
  Imot_mesure_g/1 -> Retour_états_moteur_g/2(Imot_mesure_g)
  Consigne_intensité/1 -> Retour_états_moteur_g/1(Consigne)
  Usc_mesure/1 -> Divide/2
  Divide/1 -> Saturation/1, Sum/2
  Saturation/1 -> Sum/3, Alpha_g/1, Display/1
  Retour_états_moteur_g/2(Delta_Imot_g) -> Delta_I_mot_g1/1
  Retour_états_moteur_g/3(Delta_Umot_g) -> Delta_N_mot_g1/1
  detection_saturation_correcteur1/1(correction_saturation1) -> Retour_états_moteur_g/5(anti-windup_g)
  enable/1 -> Logical Operator/1
  enable_mot_g1/1 -> Logical Operator/2
  Logical Operator/1 -> Retour_états_moteur_g/4(enable_g), Data Type Conversion/1
  Data Type Conversion/1 -> Hardware_enable_mot_1/1
  Sum/1 -> detection_saturation_correcteur1/1(saturation1)
  Saturation_alpha1/1 -> Sum/1
  Constant/1 -> Logical Operator/3
  mode/1 -> Retour_états_moteur_g/6(mode)

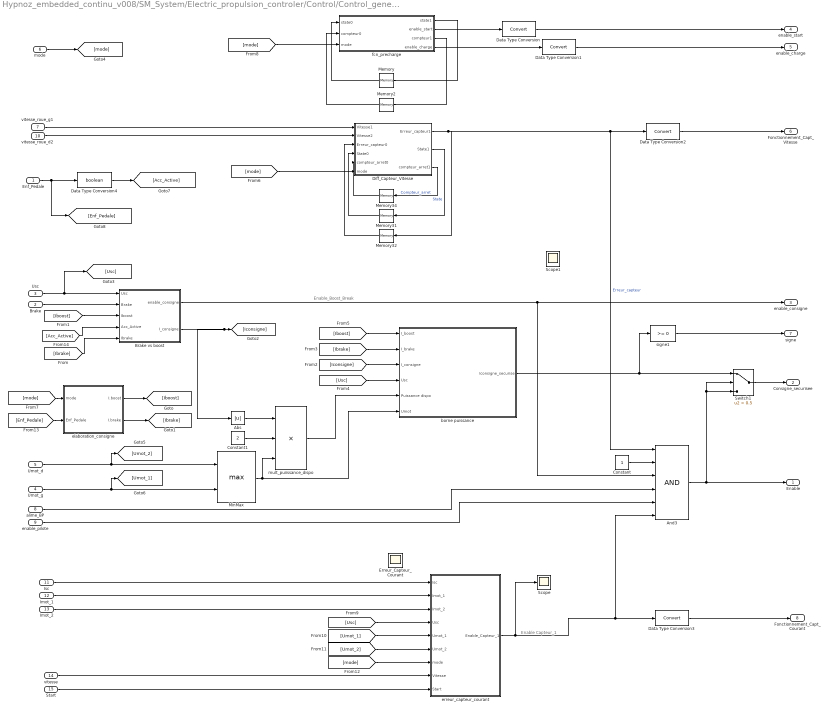
== system Hypnoz_embedded_continu_v008/SM_System/Electric_propulsion_controler/Control/Control_general_parameters ==
  note: Enable_Boost_Break
  note: Enable Capteur_1
  " Enf_Pedale" : Inport
  Brake : Inport  Port=2
  Usc : Inport  Port=3
  Umot_g : Inport  Port=4
  Umot_d : Inport  Port=5
  mode : Inport  Port=6
  vitesse_roue_g1 : Inport  Port=7
  alime_BP : Inport  Port=8
  enable_pilote : Inport  Port=9
  vitesse_roue_d2 : Inport  Port=10
  Isc : Inport  Port=11
  Imot_1 : Inport  Port=12
  Imot_2 : Inport  Port=13
  vitesse : Inport  Port=14
  Start : Inport  Port=15
  Abs : Abs
  And3 : Logic  Inputs=6  AllPortsSameDT=off  OutDataTypeStr=boolean
  Brake vs boost : Subsystem
  Constant : Constant
  Constant1 : Constant  Value=2
  Data Type Conversion{,1..3} (4 alike) : DataTypeConversion
  Data Type Conversion4 : DataTypeConversion  OutMin=[0]  OutMax=[1]  OutDataTypeStr=boolean  RndMeth=Ceiling
  Diff_Capteur_Vitesse : Stateflow chart  TreatAsAtomicUnit=on
  Erreur_Capteur_Courant : Scope  NumInputPorts=5
      settings: Floating=on  YMin=-5~-5~-5~-5~-5  YMax=5~5~5~5~5  SaveName=ScopeData2
  Memory{,2,31..32,34} (5 alike) : Memory
  MinMax : MinMax  Function=max  Inputs=2
  Scope : Scope
      settings: SaveName=ScopeData3
  Scope1 : Scope  NumInputPorts=2
      settings: YMin=-100~-1  YMax=-100~1  SaveName=ScopeData6  MaxDataPoints=50000
  Switch1 : Switch  Criteria=u2 > Threshold  Threshold=0.5
  borne puissance : Subsystem
  elaboration_consigne : Subsystem
  erreur_capteur_courant : Subsystem
  fcn_precharge : Stateflow chart  TreatAsAtomicUnit=on
  mult_puiissance_dispo : Product  Inputs=***
  signe1 : simulink/Logic and Bit Operations/Compare To Constant  SystemSampleTime=-1  relop=>=  const=0  LogicOutDataTypeMode=uint8
  Enable : Outport
  Consigne_securisee : Outport  Port=2
  enable_consigne : Outport  Port=3
  enable_start : Outport  Port=4  OutDataTypeStr=boolean
  enable_charge : Outport  Port=5  OutDataTypeStr=boolean
  Fonctionnement_Capt_Vitesse : Outport  Port=6  OutDataTypeStr=boolean
  signe : Outport  Port=7
  Fonctionnement_Capt_Courant : Outport  Port=8  OutDataTypeStr=boolean
  wires:
  Umot_g/1 -> MinMax/2, [Umot_1]
  Switch1/1 -> Consigne_securisee/1
  And3/1 -> Switch1/3, Switch1/2, Enable/1
  borne puissance/1(Iconsigne_securise) -> Switch1/1, signe1/1
  Umot_d/1 -> MinMax/1, [Umot_2]
  Abs/1 -> mult_puiissance_dispo/1
  Constant1/1 -> mult_puiissance_dispo/2
  MinMax/1 -> mult_puiissance_dispo/3, borne puissance/6(Umot)
  mult_puiissance_dispo/1 -> borne puissance/5(Puissance dispo)
  fcn_precharge/1(state1) -> Memory/1
  Memory/1 -> fcn_precharge/1(state0)
  fcn_precharge/3(compteur1) -> Memory2/1
  Memory2/1 -> fcn_precharge/2(compteur0)
  fcn_precharge/2(enable_start) -> Data Type Conversion/1
  fcn_precharge/4(enable_charge) -> Data Type Conversion1/1
  Data Type Conversion/1 -> enable_start/1
  Data Type Conversion1/1 -> enable_charge/1
  alime_BP/1 -> And3/4
  enable_pilote/1 -> And3/5
  Data Type Conversion2/1 -> Fonctionnement_Capt_Vitesse/1
  Constant/1 -> And3/2
  signe1/1 -> signe/1
  Diff_Capteur_Vitesse/3(compteur_arret1) -> Memory34/1  "Compteur_arret"
  Diff_Capteur_Vitesse/2(State1) -> Memory31/1  "State"
  Diff_Capteur_Vitesse/1(Erreur_capteur1) -> Memory32/1, Data Type Conversion2/1, And3/1  "Erreur_capteur"
  Memory34/1 -> Diff_Capteur_Vitesse/5(compteur_arret0)
  Memory31/1 -> Diff_Capteur_Vitesse/4(State0)
  Memory32/1 -> Diff_Capteur_Vitesse/3(Erreur_capteur0)
  vitesse_roue_g1/1 -> Diff_Capteur_Vitesse/1(Vitesse1)
  vitesse_roue_d2/1 -> Diff_Capteur_Vitesse/2(Vitesse2)
  Brake vs boost/2(I_consigne) -> [Iconsigne], Abs/1
  Brake vs boost/1(enable_consigne) -> enable_consigne/1, And3/3
  Usc/1 -> Brake vs boost/1(Usc), [Usc]
  Brake/1 -> Brake vs boost/2(Brake)
  [Ibrake] -> Brake vs boost/5(Ibrake)
  [Iboost] -> Brake vs boost/3(Iboost)
  [Iboost] -> borne puissance/1(I_boost)
  [Ibrake] -> borne puissance/2(I_brake)
  [Iconsigne] -> borne puissance/3(I_consigne)
  [Usc] -> borne puissance/4(Usc)
  mode/1 -> [mode]
  [mode] -> fcn_precharge/3(mode)
  [mode] -> Diff_Capteur_Vitesse/6(mode)
  [mode] -> elaboration_consigne/1(mode)
  Isc/1 -> erreur_capteur_courant/1(Isc)
  Imot_1/1 -> erreur_capteur_courant/2(Imot_1)
  Imot_2/1 -> erreur_capteur_courant/3(Imot_2)
  erreur_capteur_courant/1(Enable_Capteur_1) -> Data Type Conversion3/1, And3/6, Scope/1
  [Usc] -> erreur_capteur_courant/4(Usc)
  [Umot_1] -> erreur_capteur_courant/5(Umot_1)
  [Umot_2] -> erreur_capteur_courant/6(Umot_2)
  Data Type Conversion3/1 -> Fonctionnement_Capt_Courant/1
  [mode] -> erreur_capteur_courant/7(mode)
  vitesse/1 -> erreur_capteur_courant/8(Vitesse)
  Start/1 -> erreur_capteur_courant/9(Start)
  [Enf_Pedale] -> elaboration_consigne/2(Enf_Pedale)
  elaboration_consigne/1(I.boost) -> [Iboost]
  elaboration_consigne/2(I.brake) -> [Ibrake]
  " Enf_Pedale"/1 -> [Enf_Pedale], Data Type Conversion4/1
  Data Type Conversion4/1 -> [Acc_Active]
  [Acc_Active] -> Brake vs boost/4(Acc_Active)
  ? -> Scope1/1
  ? -> Scope1/2

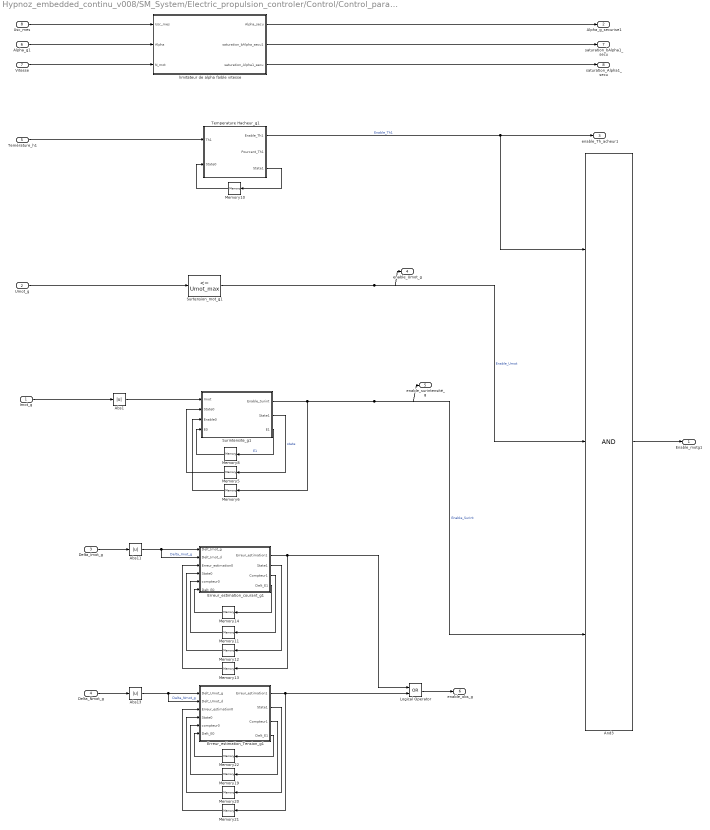
== system Hypnoz_embedded_continu_v008/SM_System/Electric_propulsion_controler/Control/Control_parameters_monitor1 ==
  Imot_g : Inport
  Umot_g : Inport  Port=2
  Delta_Imot_g : Inport  Port=3
  Delta_Nmot_g : Inport  Port=4
  Temérature_h1 : Inport  Port=5
  Alpha_g1 : Inport  Port=6
  Vitesse : Inport  Port=7
  Usc_mes : Inport  Port=8
  Abs1 : Abs
  Abs11 : Abs
  Abs13 : Abs
  And3 : Logic  Inputs=3  AllPortsSameDT=off  OutDataTypeStr=boolean
  Erreur_estimation_Tension_g1 : Stateflow chart  TreatAsAtomicUnit=on
  Erreur_estimation_courant_g1 : Stateflow chart  TreatAsAtomicUnit=on
  Logical Operator : Logic  Operator=OR  AllPortsSameDT=off  OutDataTypeStr=boolean
  Memory{5..6,8,10..14,19..22} (12 alike) : Memory
  Surintensite_g1 : Stateflow chart  TreatAsAtomicUnit=on
  Surtension_mot_g1 : simulink/Logic and Bit Operations/Compare To Constant  SystemSampleTime=-1  relop=<=  const=Umot_max  LogicOutDataTypeMode=uint8
  Temperature Hacheur_g1 : Stateflow chart  TreatAsAtomicUnit=on
  limitateur de alpha faible vitesse : Subsystem
  Enable_motg1 : Outport
  Alpha_g_securise1 : Outport  Port=2
  enable_Th_acheur1 : Outport  Port=3
  enable_Umot_g : Outport  Port=4
  enable_surintensité_g : Outport  Port=5
  enable_obs_g : Outport  Port=6
  saturation_bAlpha1_secu : Outport  Port=7
  saturation_Alpha1_secu : Outport  Port=8
  wires:
  Umot_g/1 -> Surtension_mot_g1/1
  Surtension_mot_g1/1 -> enable_Umot_g/1, And3/2  "Enable_Umot"
  And3/1 -> Enable_motg1/1
  Surintensite_g1/2(State1) -> Memory5/1  "state"
  Memory5/1 -> Surintensite_g1/2(State0)
  Memory6/1 -> Surintensite_g1/3(Enable0)
  Memory8/1 -> Surintensite_g1/4(E0)
  Surintensite_g1/1(Enable_Surint) -> Memory6/1, enable_surintensité_g/1, And3/3  "Enable_Surint"
  Surintensite_g1/3(E1) -> Memory8/1  "E1"
  Temperature Hacheur_g1/3(State1) -> Memory10/1
  Memory10/1 -> Temperature Hacheur_g1/2(State0)
  Temperature Hacheur_g1/1(Enable_Th1) -> enable_Th_acheur1/1, And3/1  "Enable_Th1"
  Erreur_estimation_courant_g1/3(Compteur1) -> Memory11/1
  Erreur_estimation_courant_g1/2(State1) -> Memory12/1
  Memory12/1 -> Erreur_estimation_courant_g1/4(State0)
  Erreur_estimation_courant_g1/4(Delt_E1) -> Memory14/1
  Memory14/1 -> Erreur_estimation_courant_g1/6(Delt_E0)
  Erreur_estimation_courant_g1/1(Erreur_estimation1) -> Memory13/1, Logical Operator/1
  Abs11/1 -> Erreur_estimation_courant_g1/1(Delt_Imot_g), Erreur_estimation_courant_g1/2(Delt_Imot_d)  "Delta_Imot_g"
  Memory13/1 -> Erreur_estimation_courant_g1/3(Erreur_estimation0)
  Memory11/1 -> Erreur_estimation_courant_g1/5(compteur0)
  Erreur_estimation_Tension_g1/3(Compteur1) -> Memory19/1
  Erreur_estimation_Tension_g1/2(State1) -> Memory20/1
  Memory20/1 -> Erreur_estimation_Tension_g1/4(State0)
  Erreur_estimation_Tension_g1/4(Delt_E1) -> Memory22/1
  Memory22/1 -> Erreur_estimation_Tension_g1/6(Delt_E0)
  Erreur_estimation_Tension_g1/1(Erreur_estimation1) -> Memory21/1, Logical Operator/2
  Abs13/1 -> Erreur_estimation_Tension_g1/1(Delt_Umot_g), Erreur_estimation_Tension_g1/2(Delt_Umot_d)  "Delta_Nmot_g"
  Memory21/1 -> Erreur_estimation_Tension_g1/3(Erreur_estimation0)
  Memory19/1 -> Erreur_estimation_Tension_g1/5(compteur0)
  Temérature_h1/1 -> Temperature Hacheur_g1/1(Th1)
  Delta_Imot_g/1 -> Abs11/1
  Delta_Nmot_g/1 -> Abs13/1
  Imot_g/1 -> Abs1/1
  Abs1/1 -> Surintensite_g1/1(Imot)
  Logical Operator/1 -> enable_obs_g/1
  Vitesse/1 -> limitateur de alpha faible vitesse/3(N_mot)
  Usc_mes/1 -> limitateur de alpha faible vitesse/1(Usc_mes)
  Alpha_g1/1 -> limitateur de alpha faible vitesse/2(Alpha)
  limitateur de alpha faible vitesse/1(Alpha_secu) -> Alpha_g_securise1/1
  limitateur de alpha faible vitesse/2(saturation_bAlpha_secu1) -> saturation_bAlpha1_secu/1
  limitateur de alpha faible vitesse/3(saturation_Alpha1_secu) -> saturation_Alpha1_secu/1

== system Hypnoz_embedded_continu_v008/SM_System/Modele_Physique_Voiture_Simple/Circuit_electrique_HP/Moteur_electrique_d ==
  TensionSortieHacheur : Inport
  Vitesse : Inport  Port=2
  Add3 : Sum  Inputs=+-
  Gain2 : Gain  Gain=k
  Zero-Pole : ZeroPole  Zeros=[]  Poles=[-r/L]  Gain=[1/L]
  CourantMoteur : Outport
  wires:
  Add3/1 -> Zero-Pole/1
  Zero-Pole/1 -> CourantMoteur/1
  TensionSortieHacheur/1 -> Add3/1
  Vitesse/1 -> Gain2/1
  Gain2/1 -> Add3/2

== system Hypnoz_embedded_continu_v008/SM_System/Modele_Physique_Voiture_Simple/Circuit_electrique_HP/Moteur_electrique_g ==
  TensionSortieHacheur : Inport
  Vitesse : Inport  Port=2
  Add3 : Sum  Inputs=+-
  Gain2 : Gain  Gain=k
  Zero-Pole : ZeroPole  Zeros=[]  Poles=[-r/L]  Gain=[1/L]
  CourantMoteur : Outport
  wires:
  Add3/1 -> Zero-Pole/1
  Zero-Pole/1 -> CourantMoteur/1
  TensionSortieHacheur/1 -> Add3/1
  Vitesse/1 -> Gain2/1
  Gain2/1 -> Add3/2

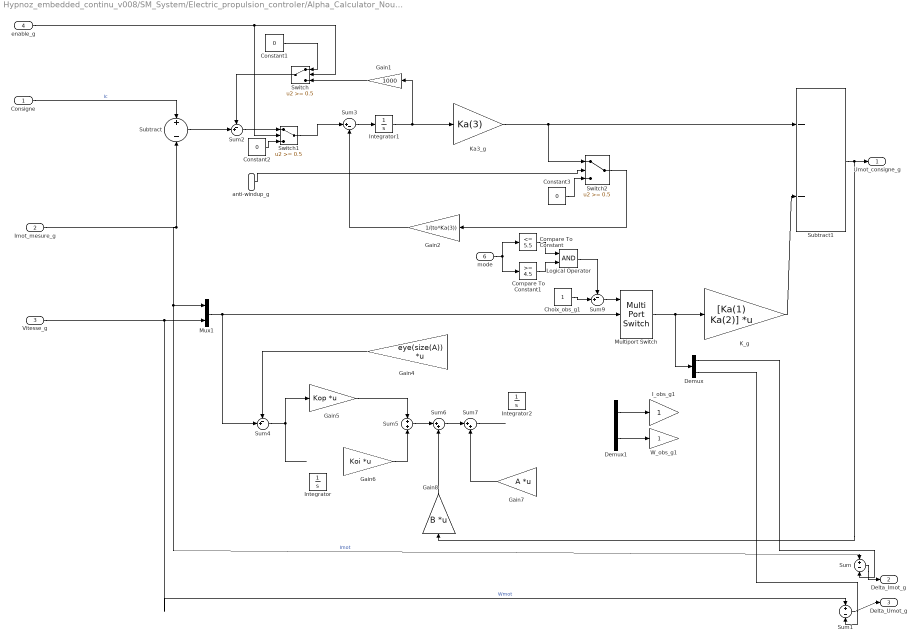
== system Hypnoz_embedded_continu_v008/SM_System/Electric_propulsion_controler/Alpha_Calculator_Nouveau/Alpha_calculator_motg1/Retour_états_moteur_g ==
  Consigne : Inport
  Imot_mesure_g : Inport  Port=2
  Vitesse_g : Inport  Port=3
  enable_g : Inport  Port=4
  anti-windup_g : Inport  Port=5
  mode : Inport  Port=6
  Choix_obs_g1 : Constant
  Compare To Constant : simulink/Logic and Bit Operations/Compare To Constant  SystemSampleTime=-1  relop=<=  const=5.5  LogicOutDataTypeMode=uint8
  Compare To Constant1 : simulink/Logic and Bit Operations/Compare To Constant  SystemSampleTime=-1  relop=>=  const=4.5  LogicOutDataTypeMode=uint8
  Constant1 : Constant  Value=0
  Constant2 : Constant  Value=0
  Constant3 : Constant  Value=0
  Demux : Demux  Outputs=2
  Demux1 : Demux  Outputs=2
  Gain1 : Gain  Gain=1000
  Gain2 : Gain  Gain=1/(to*Ka(3))
  Gain4 : Gain  Gain=eye(size(A))  Multiplication=Matrix(K*u) (u vector)
  Gain5 : Gain  Gain=Kop  Multiplication=Matrix(K*u) (u vector)
  Gain6 : Gain  Gain=Koi  Multiplication=Matrix(K*u) (u vector)
  Gain7 : Gain  Gain=A  Multiplication=Matrix(K*u) (u vector)
  Gain8 : Gain  Gain=B  Multiplication=Matrix(K*u) (u vector)
  I_obs_g1 : Gain
  Integrator : Integrator
  Integrator1 : Integrator
  Integrator2 : Integrator
  K_g : Gain  Gain=[Ka(1) Ka(2)]  Multiplication=Matrix(K*u) (u vector)
  Ka3_g : Gain  Gain=Ka(3)
  Logical Operator : Logic  AllPortsSameDT=off  OutDataTypeStr=boolean
  Multiport Switch : MultiPortSwitch  Inputs=2  zeroidx=off
  Mux1 : Mux  Inputs=2
  Subtract : Sum  Inputs=+-  SampleTime=Ts
  Subtract1 : Sum  Inputs=--
  Sum : Sum  Inputs=+|-
  Sum1 : Sum  Inputs=+|-
  Sum2 : Sum  Inputs=-+|
  Sum3 : Sum  Inputs=|+-
  Sum4 : Sum  Inputs=-+|
  Sum5 : Sum  Inputs=+|+
  Sum6 : Sum  Inputs=|++
  Sum7 : Sum  Inputs=|++
  Sum9 : Sum  Inputs=-+|
  Switch : Switch  Threshold=0.5
  Switch1 : Switch  Threshold=0.5
  Switch2 : Switch  Threshold=0.5
  W_obs_g1 : Gain
  Umot_consigne_g : Outport
  Delta_Imot_g : Outport  Port=2
  Delta_Umot_g : Outport  Port=3
  wires:
  Imot_mesure_g/1 -> Subtract/2, Sum/1, Mux1/1  "Imot"
  Consigne/1 -> Subtract/1  "Ic"
  Ka3_g/1 -> Subtract1/1, Switch2/1
  Subtract1/1 -> Umot_consigne_g/1, Gain8/1
  K_g/1 -> Subtract1/2
  Vitesse_g/1 -> Sum1/1, Mux1/2  "Wmot"
  Integrator1/1 -> Gain1/1, Ka3_g/1
  Subtract/1 -> Sum2/2
  Sum3/1 -> Integrator1/1
  Switch2/1 -> Gain2/1
  Constant3/1 -> Switch2/3
  anti-windup_g/1 -> Switch2/2
  Gain2/1 -> Sum3/2
  enable_g/1 -> Switch/2, Switch1/2
  Gain1/1 -> Switch/3
  Switch/1 -> Sum2/1
  Constant1/1 -> Switch/1
  Sum/1 -> Delta_Imot_g/1
  Sum1/1 -> Delta_Umot_g/1
  Demux/1 -> Sum/2
  Demux/2 -> Sum1/2
  Mux1/1 -> Multiport Switch/2, Sum4/2
  Multiport Switch/1 -> K_g/1, Demux/1
  ? -> Gain6/1
  Sum4/1 -> Gain5/1
  Gain6/1 -> Sum5/2
  Gain5/1 -> Sum5/1
  Sum5/1 -> Sum6/1
  Gain8/1 -> Sum6/2
  Sum6/1 -> Sum7/1
  Sum7/1 -> ?
  Gain7/1 -> Sum7/2
  ? -> Gain7/1, Gain4/1, Multiport Switch/3, Demux1/1
  Gain4/1 -> Sum4/1
  Demux1/1 -> I_obs_g1/1
  Demux1/2 -> W_obs_g1/1
  Sum2/1 -> Switch1/1
  Switch1/1 -> Sum3/1
  Constant2/1 -> Switch1/3
  Choix_obs_g1/1 -> Sum9/2
  mode/1 -> Compare To Constant/1, Compare To Constant1/1
  Compare To Constant/1 -> Logical Operator/1
  Compare To Constant1/1 -> Logical Operator/2
  Logical Operator/1 -> Sum9/1
  Sum9/1 -> Multiport Switch/1

== system Hypnoz_embedded_continu_v008/SM_System/Electric_propulsion_controler/Alpha_Calculator_Nouveau/Alpha_calculator_motg1/detection_saturation_correcteur1 ==
  saturation1 : Inport
  Compare To Constant : simulink/Logic and Bit Operations/Compare To Constant  SystemSampleTime=-1  relop=>=  const=0.01  LogicOutDataTypeMode=uint8
  Constant1 : Constant  Value=0
  Switch : Switch  Threshold=0.5
  correction_saturation1 : Outport
  wires:
  saturation1/1 -> Switch/1, Compare To Constant/1
  Compare To Constant/1 -> Switch/2
  Constant1/1 -> Switch/3
  Switch/1 -> correction_saturation1/1

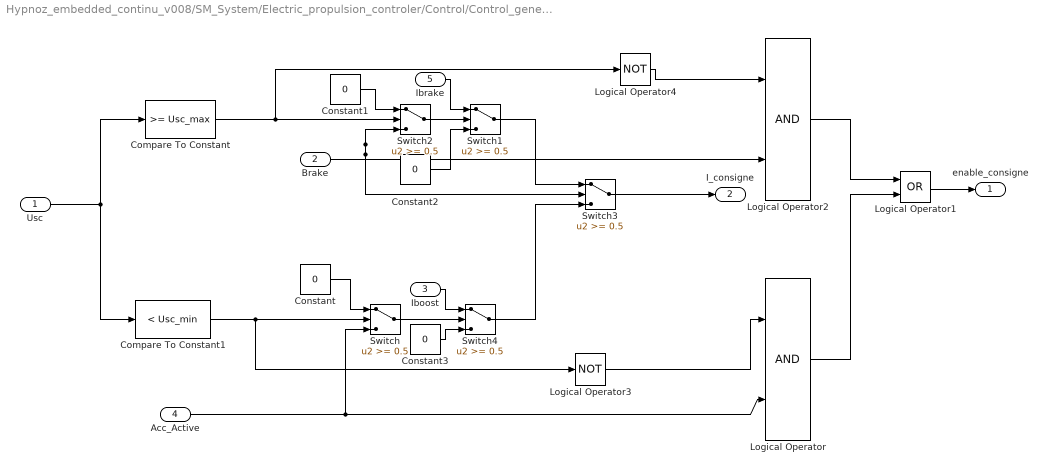
== system Hypnoz_embedded_continu_v008/SM_System/Electric_propulsion_controler/Control/Control_general_parameters/Brake vs boost ==
  Usc : Inport
  Brake : Inport  Port=2
  Iboost : Inport  Port=3
  Acc_Active : Inport  Port=4
  Ibrake : Inport  Port=5
  Compare To Constant : simulink/Logic and Bit Operations/Compare To Constant  SystemSampleTime=-1  relop=>=  const=Usc_max  LogicOutDataTypeMode=uint8
  Compare To Constant1 : simulink/Logic and Bit Operations/Compare To Constant  SystemSampleTime=-1  relop=<  const=Usc_min  LogicOutDataTypeMode=uint8
  Constant{,1..3} (4 alike) : Constant  Value=0
  Logical Operator : Logic  AllPortsSameDT=off  OutDataTypeStr=boolean
  Logical Operator1 : Logic  Operator=OR  AllPortsSameDT=off  OutDataTypeStr=boolean
  Logical Operator2 : Logic  AllPortsSameDT=off  OutDataTypeStr=boolean
  Logical Operator3 : Logic  Operator=NOT  AllPortsSameDT=off  OutDataTypeStr=boolean
  Logical Operator4 : Logic  Operator=NOT  AllPortsSameDT=off  OutDataTypeStr=boolean
  Switch{,1..4} (5 alike) : Switch  Threshold=0.5
  enable_consigne : Outport
  I_consigne : Outport  Port=2
  wires:
  Usc/1 -> Compare To Constant/1, Compare To Constant1/1
  Compare To Constant/1 -> Switch2/2, Logical Operator4/1
  Compare To Constant1/1 -> Switch/2, Logical Operator3/1
  Constant/1 -> Switch/1
  Constant1/1 -> Switch2/1
  Constant3/1 -> Switch4/3
  Brake/1 -> Switch2/3, Switch3/2, Logical Operator2/2
  Switch2/1 -> Switch1/2
  Constant2/1 -> Switch1/3
  Switch/1 -> Switch4/2
  Acc_Active/1 -> Switch/3, Logical Operator/2
  Iboost/1 -> Switch4/1
  Ibrake/1 -> Switch1/1
  Switch4/1 -> Switch3/3
  Switch1/1 -> Switch3/1
  Switch3/1 -> I_consigne/1
  Logical Operator2/1 -> Logical Operator1/1
  Logical Operator/1 -> Logical Operator1/2
  Logical Operator1/1 -> enable_consigne/1
  Logical Operator3/1 -> Logical Operator/1
  Logical Operator4/1 -> Logical Operator2/1

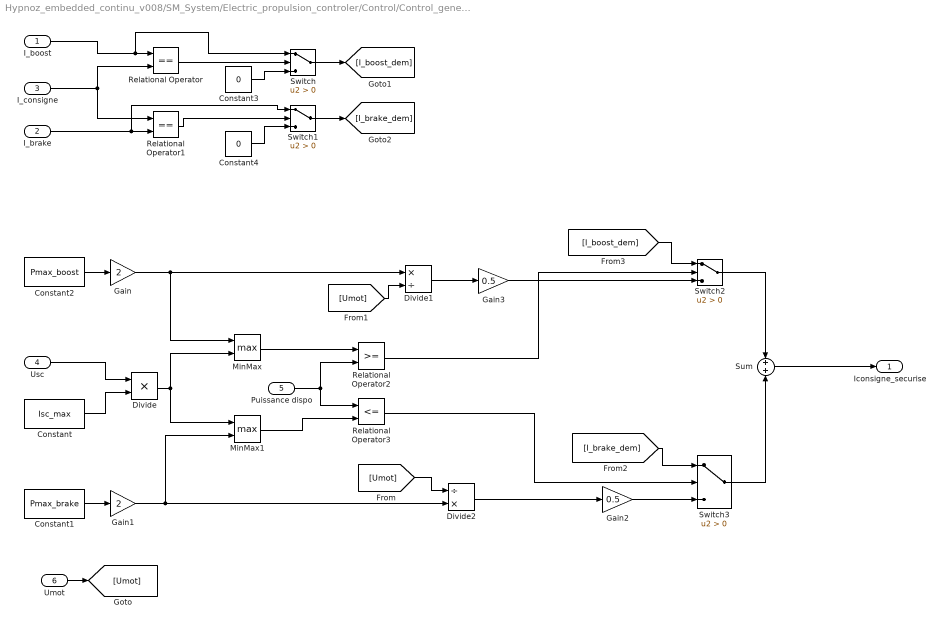
== system Hypnoz_embedded_continu_v008/SM_System/Electric_propulsion_controler/Control/Control_general_parameters/borne puissance ==
  I_boost : Inport
  I_brake : Inport  Port=2
  I_consigne : Inport  Port=3
  Usc : Inport  Port=4
  Puissance dispo : Inport  Port=5
  Umot : Inport  Port=6
  Constant : Constant  Value=Isc_max
  Constant1 : Constant  Value=Pmax_brake
  Constant2 : Constant  Value=Pmax_boost
  Constant3 : Constant  Value=0
  Constant4 : Constant  Value=0
  Divide : Product  Inputs=**
  Divide1 : Product  Inputs=*/
  Divide2 : Product  Inputs=/*
  Gain : Gain  Gain=2
  Gain1 : Gain  Gain=2
  Gain2 : Gain  Gain=0.5
  Gain3 : Gain  Gain=0.5
  MinMax : MinMax  Function=max  Inputs=2
  MinMax1 : MinMax  Function=max  Inputs=2
  Relational Operator : RelationalOperator  Operator===  OutDataTypeStr=boolean
  Relational Operator1 : RelationalOperator  Operator===  OutDataTypeStr=boolean
  Relational Operator2 : RelationalOperator  OutDataTypeStr=boolean
  Relational Operator3 : RelationalOperator  Operator=<=  OutDataTypeStr=boolean
  Sum : Sum  Inputs=+|+
  Switch{,1..3} (4 alike) : Switch  Criteria=u2 > Threshold
  Iconsigne_securise : Outport
  wires:
  I_boost/1 -> Relational Operator/1, Switch/1
  I_consigne/1 -> Relational Operator/2, Relational Operator1/1
  Usc/1 -> Divide/1
  Constant/1 -> Divide/2
  I_brake/1 -> Relational Operator1/2, Switch1/1
  Constant2/1 -> Gain/1
  Gain/1 -> MinMax/1, Divide1/1
  Divide/1 -> MinMax/2, MinMax1/1
  Constant1/1 -> Gain1/1
  Gain1/1 -> MinMax1/2, Divide2/2
  MinMax/1 -> Relational Operator2/1
  Puissance dispo/1 -> Relational Operator2/2, Relational Operator3/1
  MinMax1/1 -> Relational Operator3/2
  Relational Operator/1 -> Switch/2
  Constant3/1 -> Switch/3
  Constant4/1 -> Switch1/3
  Relational Operator1/1 -> Switch1/2
  Relational Operator2/1 -> Switch2/2
  Divide1/1 -> Gain3/1
  Divide2/1 -> Gain2/1
  Gain2/1 -> Switch3/3
  Relational Operator3/1 -> Switch3/2
  Switch2/1 -> Sum/1
  Switch3/1 -> Sum/2
  Sum/1 -> Iconsigne_securise/1
  Gain3/1 -> Switch2/3
  Umot/1 -> [Umot]
  [Umot] -> Divide1/2
  [Umot] -> Divide2/1
  Switch/1 -> [I_boost_dem]
  Switch1/1 -> [I_brake_dem]
  [I_boost_dem] -> Switch2/1
  [I_brake_dem] -> Switch3/1

== system Hypnoz_embedded_continu_v008/SM_System/Electric_propulsion_controler/Control/Control_general_parameters/elaboration_consigne ==
  mode : Inport
  Enf_Pedale : Inport  Port=2
  1 : Constant  Value=200
  2 : Constant  Value=200
  3 : Constant  Value=-200
  4 : Constant  Value=100
  5 : Constant  Value=200
  Constant2 : Constant  Value=0
  Constant3 : Constant  Value=-100
  Constant4 : Constant  Value=-250
  Courant Acceleration : MultiPortSwitch  Inputs=5  zeroidx=off  RndMeth=Nearest
  Courant Brake : MultiPortSwitch  Inputs=5  zeroidx=off  RndMeth=Nearest
  I_boost : Constant  Value=200
  I_brake : Constant  Value=0
  Model Info : simulink/Model-Wide Utilities/Model Info  SystemSampleTime=-1  InitialBlockCM=None  BlockCM=None  Frame=on  DisplayStringWithTags=|  HorizontalTextAlignment=Center  LeftAlignmentValue=0.5  SourceBlockDiagram=Hypnoz_embedded_continu_v008  TagMaxNumber=20
      | Description des Modes
      | Mode 1: Normal
      | Mode 2: Intensités Réduites
      | Mode 3: Sans Récuperatif
      | Mode 4: Boost (Binaire)
      | Mode 5: Boost Sans Récuperatif
  Product : Product  RndMeth=Zero
  Product1 : Product  RndMeth=Zero
  Product2 : Product  RndMeth=Zero
  I.boost : Outport
  I.brake : Outport  Port=2
  wires:
  I_boost/1 -> Courant Acceleration/6
  2/1 -> Courant Acceleration/5
  Enf_Pedale/1 -> Product/2, Product1/2, Product2/2
  Product/1 -> Courant Acceleration/4
  1/1 -> Product/1
  Product1/1 -> Courant Acceleration/3
  4/1 -> Product1/1
  Product2/1 -> Courant Acceleration/2
  5/1 -> Product2/1
  Courant Acceleration/1 -> I.boost/1
  mode/1 -> Courant Acceleration/1, Courant Brake/1
  Courant Brake/1 -> I.brake/1
  I_brake/1 -> Courant Brake/6
  3/1 -> Courant Brake/5
  Constant2/1 -> Courant Brake/4
  Constant3/1 -> Courant Brake/3
  Constant4/1 -> Courant Brake/2

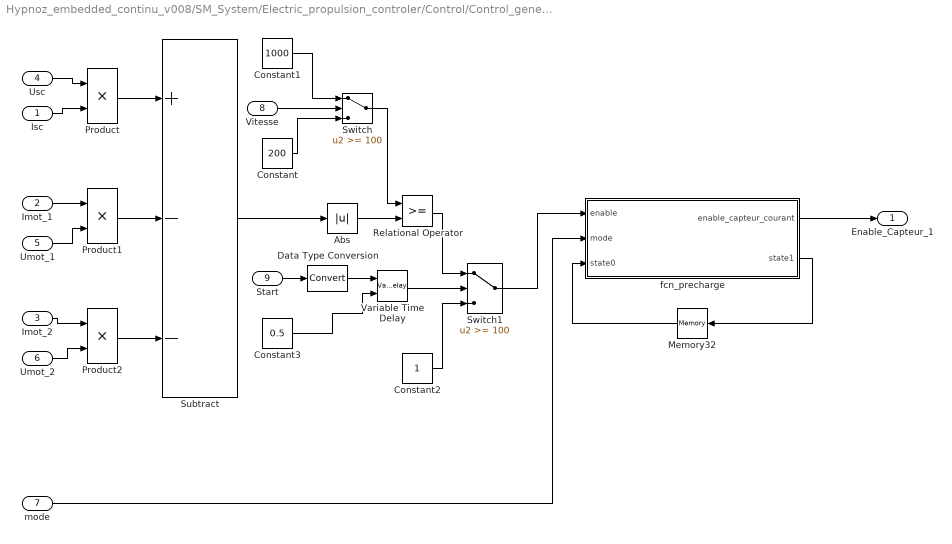
== system Hypnoz_embedded_continu_v008/SM_System/Electric_propulsion_controler/Control/Control_general_parameters/erreur_capteur_courant ==
  Isc : Inport
  Imot_1 : Inport  Port=2
  Imot_2 : Inport  Port=3
  Usc : Inport  Port=4
  Umot_1 : Inport  Port=5
  Umot_2 : Inport  Port=6
  mode : Inport  Port=7
  Vitesse : Inport  Port=8
  Start : Inport  Port=9
  Abs : Abs
  Constant : Constant  Value=200
  Constant1 : Constant  Value=1000
  Constant2 : Constant
  Constant3 : Constant  Value=0.5
  Data Type Conversion : DataTypeConversion
  Memory32 : Memory
  Product : Product  RndMeth=Zero
  Product1 : Product  RndMeth=Zero
  Product2 : Product  RndMeth=Zero
  Relational Operator : RelationalOperator  OutDataTypeStr=boolean
  Subtract : Sum  Inputs=+--
  Switch : Switch  Threshold=100
  Switch1 : Switch  Threshold=100
  Variable Time Delay : VariableTransportDelay
  fcn_precharge : Stateflow chart  TreatAsAtomicUnit=on
  Enable_Capteur_1 : Outport
  wires:
  Subtract/1 -> Abs/1
  Usc/1 -> Product/1
  Isc/1 -> Product/2
  Imot_1/1 -> Product1/1
  Umot_1/1 -> Product1/2
  Imot_2/1 -> Product2/1
  Umot_2/1 -> Product2/2
  Product/1 -> Subtract/1
  Product1/1 -> Subtract/2
  Product2/1 -> Subtract/3
  fcn_precharge/1(enable_capteur_courant) -> Enable_Capteur_1/1
  mode/1 -> fcn_precharge/2(mode)
  fcn_precharge/2(state1) -> Memory32/1
  Memory32/1 -> fcn_precharge/3(state0)
  Constant/1 -> Switch/3
  Constant1/1 -> Switch/1
  Vitesse/1 -> Switch/2
  Abs/1 -> Relational Operator/2
  Switch/1 -> Relational Operator/1
  Switch1/1 -> fcn_precharge/1(enable)
  Relational Operator/1 -> Switch1/1
  Constant2/1 -> Switch1/3
  Start/1 -> Data Type Conversion/1
  Variable Time Delay/1 -> Switch1/2
  Constant3/1 -> Variable Time Delay/2
  Data Type Conversion/1 -> Variable Time Delay/1

== system Hypnoz_embedded_continu_v008/SM_System/Electric_propulsion_controler/Control/Control_parameters_monitor1/limitateur de alpha faible vitesse ==
  Usc_mes : Inport
  Alpha : Inport  Port=2
  N_mot : Inport  Port=3
  Compare To Constant : simulink/Logic and Bit Operations/Compare To Constant  SystemSampleTime=-1  relop=<=  const=300  LogicOutDataTypeMode=uint8
  Compare To Constant1 : simulink/Logic and Bit Operations/Compare To Constant  SystemSampleTime=-1  relop=>=  const=35  LogicOutDataTypeMode=uint8
  Constant : Constant  Value=25
  Divide : Product  Inputs=**
  Divide1 : Product  Inputs=*/
  Logical Operator1 : Logic  AllPortsSameDT=off  OutDataTypeStr=boolean
  Sum : Sum  Inputs=+|-
  Switch : Switch  Threshold=0.5  OutDataTypeStr=Inherit: Inherit via back propagation
  Alpha_secu : Outport
  saturation_bAlpha_secu1 : Outport  Port=2
  saturation_Alpha1_secu : Outport  Port=3
  wires:
  Usc_mes/1 -> Divide/1, Divide1/2
  Alpha/1 -> Divide/2, Switch/3, Sum/1
  Divide/1 -> Compare To Constant1/1
  Compare To Constant1/1 -> Logical Operator1/1
  Compare To Constant/1 -> Logical Operator1/2
  Logical Operator1/1 -> Switch/2, saturation_bAlpha_secu1/1
  Divide1/1 -> Switch/1
  Constant/1 -> Divide1/1
  Switch/1 -> Alpha_secu/1, Sum/2
  N_mot/1 -> Compare To Constant/1
  Sum/1 -> saturation_Alpha1_secu/1
